simulink model "system1_net"  (R2019b)
settings: Solver=VariableStepAuto  StartTime=0.0  StopTime=10.0  RelTol=1e-3
settings Model: Creator=davis  LastModifiedBy=davis

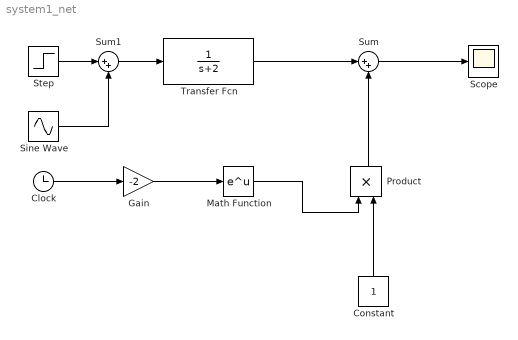
== system system1_net ==
  Clock : Clock
  Constant : Constant
  Gain : Gain  Gain=-2
  Math Function : Math  SignedPower=off  SaturateOnIntegerOverflow=on
  Product : Product
  Scope : Scope
  Sine Wave : Sin  SampleTime=0
  Step : Step  Time=0  SampleTime=0
  Sum : Sum  Inputs=|++
  Sum1 : Sum  Inputs=|++
  Transfer Fcn : TransferFcn  Denominator=[1 2]
  wires:
  Transfer Fcn/1 -> Sum/1
  Product/1 -> Sum/2
  Clock/1 -> Gain/1
  Gain/1 -> Math Function/1
  Math Function/1 -> Product/1
  Constant/1 -> Product/2
  Sum/1 -> Scope/1
  Step/1 -> Sum1/1
  Sum1/1 -> Transfer Fcn/1
  Sine Wave/1 -> Sum1/2
